simulink model "Aeropendulum"  (R2016b)
settings: Solver=VariableStepAuto  StartTime=0.0  StopTime=10.0  RelTol=1e-3
model workspace (MAT data in the model file):
  P_Gain = 0.0555555555556
  a_gravity = 9.81
  air_den = 1.225
  diam_prop = 3.1
  m_Motor = 1
  v_air = 0
  v_prop = 6000
  volt_max = 5
settings Model: Creator=Joseph  LastModifiedBy=Joseph

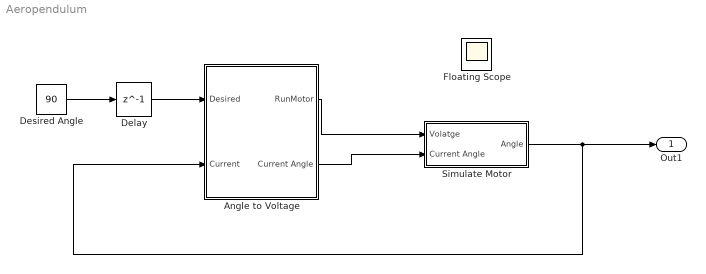
== system Aeropendulum ==
  Angle to Voltage : Subsystem
  Delay : Delay  DelayLength=1  InitialCondition=0
  "Desired Angle " : Constant  Value=90
  Floating Scope : Scope
      settings: Floating=on
  Simulate Motor : Subsystem
  Out1 : Outport
  wires:
  "Desired Angle "/1 -> Delay/1
  Simulate Motor/1(Angle) -> Angle to Voltage/2(Current), Out1/1
  Angle to Voltage/1(RunMotor) -> Simulate Motor/1(Volatge)
  Angle to Voltage/2("Current Angle ") -> Simulate Motor/2(Current Angle)
  Delay/1 -> Angle to Voltage/1("Desired ")

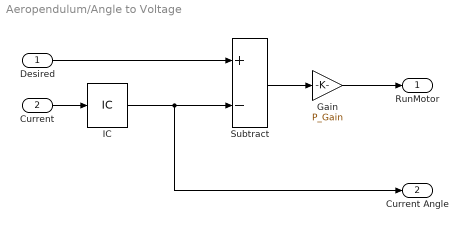
== system Aeropendulum/Angle to Voltage ==
  "Desired " : Inport
  Current : Inport  Port=2
  Gain : Gain  Gain=P_Gain
  IC : InitialCondition  Value=0
  Subtract : Sum  Inputs=+-
  RunMotor : Outport
  "Current Angle " : Outport  Port=2
  wires:
  Subtract/1 -> Gain/1
  "Desired "/1 -> Subtract/1
  Gain/1 -> RunMotor/1
  Current/1 -> IC/1
  IC/1 -> "Current Angle "/1, Subtract/2

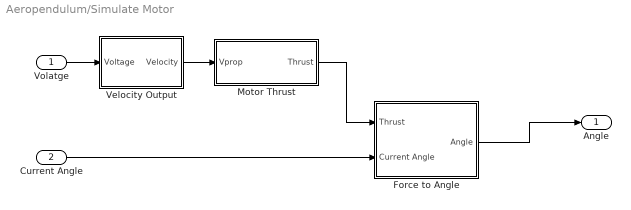
== system Aeropendulum/Simulate Motor ==
  Volatge : Inport
  Current Angle : Inport  Port=2
  Force to Angle : Subsystem
  Motor Thrust : Subsystem
  "Velocity Output " : Subsystem
  Angle : Outport
  wires:
  Volatge/1 -> "Velocity Output "/1(Voltage)
  "Velocity Output "/1(Velocity) -> Motor Thrust/1(Vprop)
  Force to Angle/1(Angle) -> Angle/1
  Motor Thrust/1(Thrust) -> Force to Angle/1(Thrust)
  Current Angle/1 -> Force to Angle/2(Current Angle)

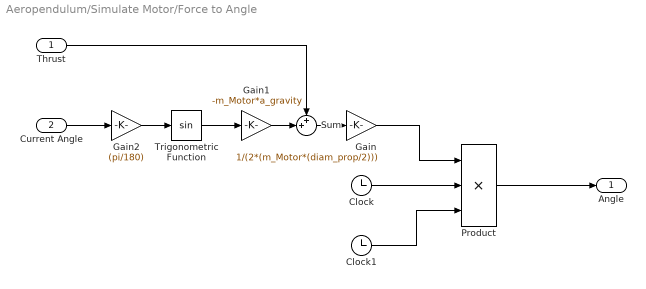
== system Aeropendulum/Simulate Motor/Force to Angle ==
  Thrust : Inport
  Current Angle : Inport  Port=2
  Clock : Clock
  Clock1 : Clock
  Gain : Gain  Gain=1/(2*(m_Motor*(diam_prop/2)))
  Gain1 : Gain  Gain=-m_Motor*a_gravity
  Gain2 : Gain  Gain=(pi/180)
  Product : Product  Inputs=3
  Sum : Sum  Inputs=++|
  Trigonometric Function : Trigonometry
  Angle : Outport
  wires:
  Trigonometric Function/1 -> Gain1/1
  Thrust/1 -> Sum/1
  Gain1/1 -> Sum/2
  Sum/1 -> Gain/1
  Clock/1 -> Product/2
  Gain/1 -> Product/1
  Clock1/1 -> Product/3
  Product/1 -> Angle/1
  Current Angle/1 -> Gain2/1
  Gain2/1 -> Trigonometric Function/1

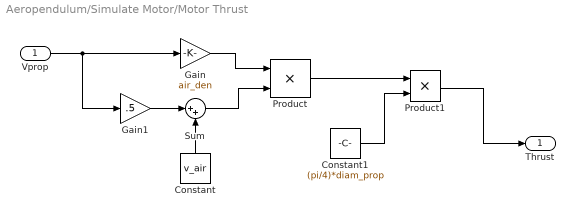
== system Aeropendulum/Simulate Motor/Motor Thrust ==
  Vprop : Inport
  Constant : Constant  Value=v_air
  Constant1 : Constant  Value=(pi/4)*diam_prop
  Gain : Gain  Gain=air_den
  Gain1 : Gain  Gain=.5
  Product : Product
  Product1 : Product
  Sum : Sum  Inputs=|++
  Thrust : Outport
  wires:
  Vprop/1 -> Gain1/1, Gain/1
  Constant/1 -> Sum/2
  Gain1/1 -> Sum/1
  Sum/1 -> Product/2
  Gain/1 -> Product/1
  Product/1 -> Product1/1
  Constant1/1 -> Product1/2
  Product1/1 -> Thrust/1

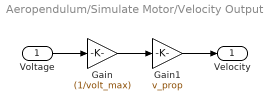
== system Aeropendulum/Simulate Motor/Velocity Output  ==
  Voltage : Inport
  Gain : Gain  Gain=(1/volt_max)
  Gain1 : Gain  Gain=v_prop
  Velocity : Outport
  wires:
  Voltage/1 -> Gain/1
  Gain/1 -> Gain1/1
  Gain1/1 -> Velocity/1
